simulink model "untitled"  (R2018b)
settings: Solver=VariableStepAuto  StartTime=0.0  StopTime=1  RelTol=1e-3
settings Model: Creator=70654  LastModifiedBy=70654
settings DataIOCC: ReturnWorkspaceOutputs=on

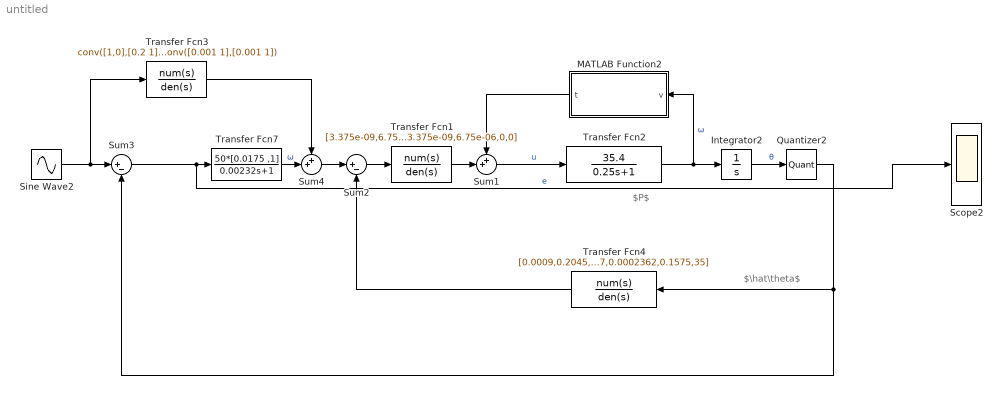
== system untitled ==
  note: $\hat\theta$
  note: $P$
  Integrator2 : Integrator
  MATLAB Function2 : MATLAB Function  TreatAsAtomicUnit=on
  Quantizer2 : Quantizer  QuantizationInterval=1/1800
  Scope2 : Scope  NumInputPorts=3
  Sine Wave2 : Sin  Amplitude=0.5  Frequency=10*2*pi  SampleTime=0
  Sum1 : Sum  Inputs=++|
  Sum2 : Sum  Inputs=|+-
  Sum3 : Sum  Inputs=|+-
  Sum4 : Sum  Inputs=++|
  Transfer Fcn1 : TransferFcn  Numerator=[3.375e-09,6.75e-06,0.0045,1]  Denominator=[3.375e-09,6.75e-06,0,0]
  Transfer Fcn2 : TransferFcn  Numerator=[35.4]  Denominator=[0.25 1]
  Transfer Fcn3 : TransferFcn  Numerator=conv([1,0],[0.2 1])  Denominator=35*conv([0.001 1],[0.001 1])
  Transfer Fcn4 : TransferFcn  Numerator=[0.0009,0.2045,1,0]  Denominator=[1.181e-07,0.0002362,0.1575,35]
  Transfer Fcn7 : TransferFcn  Numerator=50*[0.0175 ,1]  Denominator=[0.00232,1]
  wires:
  Transfer Fcn2/1 -> Integrator2/1, MATLAB Function2/1(v)  "ω"
  Sum3/1 -> Scope2/2, Transfer Fcn7/1  "e"
  Integrator2/1 -> Quantizer2/1  "θ"
  Quantizer2/1 -> Transfer Fcn4/1, Sum3/2
  Sum1/1 -> Transfer Fcn2/1  "u"
  Sine Wave2/1 -> Transfer Fcn3/1, Sum3/1
  Sum2/1 -> Transfer Fcn1/1
  Transfer Fcn1/1 -> Sum1/2
  MATLAB Function2/1(t) -> Sum1/1
  Transfer Fcn4/1 -> Sum2/2
  Transfer Fcn7/1 -> Sum4/2  "ω"
  Sum4/1 -> Sum2/1
  Transfer Fcn3/1 -> Sum4/1

== matlab function untitled/MATLAB Function2 ==
  data: v input; t output
function t = fcn(v)
t = 0.8*v + (1 + 9*exp(-2.2*abs(v)))*sign(v);
end
